simulink model "FlightCore_Gazebo_loop"  (R2025b)
settings: Solver=FixedStepDiscrete  StartTime=0.0  StopTime=(double(GazeboLockstepEpochCount)-1)*GazeboLockstepSampleTime  FixedStep=GazeboLockstepSampleTime  RelTol=1e-3
model workspace (MAT data in the model file):
  GazeboLockstepEpochCount = 20
  GazeboLockstepSampleTime = 0.001
  GazeboLockstepSessionId = 1167057969
  GazeboPrimeTimeoutSec = 300
  GazeboStepResultTimeoutSec = 5
  SL_Bus_ROSEnable64bitIntegers = 1
undefined symbols (not defined in the file): actuator_values, armed, command_id, source_step_id, target_step_id, valid, valid_from_iteration
libraries: ros2lib x4
settings Model: DataDictionary=GlobalTypes.sldd  PacingRate=0.250000  Creator=89447  LastModifiedBy=89447
settings OptimizationCC: DefaultParameterBehavior=Inlined  EnhancedBackFolding=on  PassReuseOutputArgsAs=Individual arguments  ZeroExternalMemoryAtStartup=off  ZeroInternalMemoryAtStartup=off  MaxStackSize=64  OptimizeBlockOrder=speed  DifferentSizesBufferReuse=on  OptimizationCustomize=off  EfficientTunableParamExpr=on
settings HardwareCC: ProdBitPerLong=64.0  ProdHWDeviceType=Intel->x86-64 (Linux 64)
settings SFSimCC: MATLABDynamicMemAlloc=off
settings RTWCC: SystemTargetFile=ert.tlc  HardwareBoard=Robot Operating System 2 (ROS 2)  TLCOptions="-aInlineSetEventsForThisBaseRateFcn=TLC_FALSE -aSuppressMultiTaskScheduler=TLC_FALSE  -aRateBasedStepFcn=0"  GenCodeOnly=on  TemplateMakefile=ert_default_tmf  Toolchain=Colcon Tools  TargetLang=C++  Description=Embedded Coder
settings CodeAppCC: ForceParamTrailComments=on  IgnoreCustomStorageClasses=off  OperatorAnnotations=on  SimulinkDataObjDesc=on  SFDataObjDesc=on  InsertBlockDesc=on
settings ERTTargetCC: ExtModeTransport=2.0  ExtModeStaticAlloc=on  ExtModeAutomaticAllocSize=off  ExtModeMexFile=ext_xcp  ExtModeIntrfLevel=Level2 - Open  RootIOFormat=Structure reference  TargetLangStandard=C++11 (ISO)  CodeInterfacePackaging=C++ class  SupportContinuousTime=on

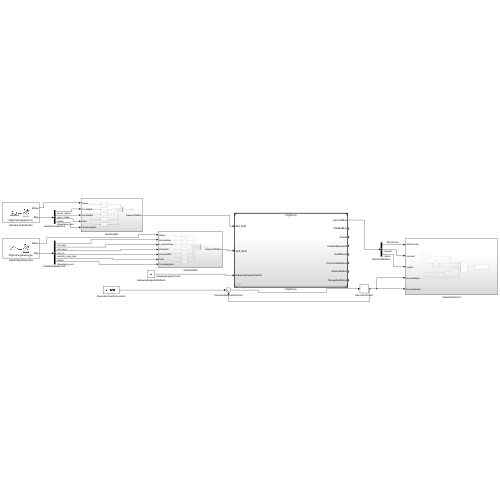
[thumbnail: Simulink's stored preview of the top-level diagram]
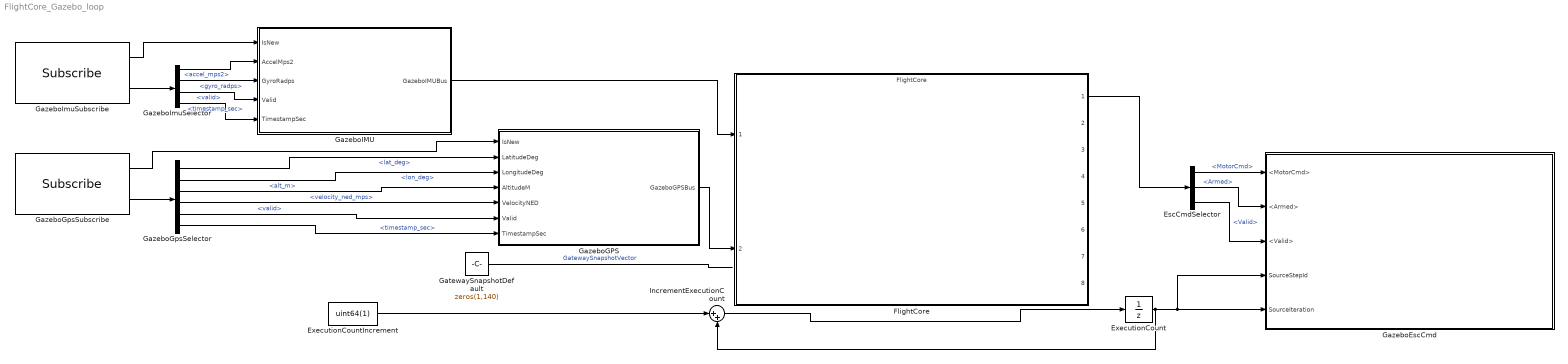
== system FlightCore_Gazebo_loop ==
  EscCmdSelector : BusSelector  OutputSignals=MotorCmd,Armed,Valid
  ExecutionCount : UnitDelay  InitialCondition=uint64(0)  SampleTime=GazeboLockstepSampleTime
  ExecutionCountIncrement : Constant  Value=uint64(1)  SampleTime=GazeboLockstepSampleTime
  FlightCore : ModelReference  ModelNameDialog=FlightCore  SimulationMode=Normal  ModelReferenceVersion=1.37
  GatewaySnapshotDefault : Constant  Value=zeros(1,140)  OutDataTypeStr=double  SampleTime=-1
  GazeboEscCmd : Subsystem
  GazeboGPS : Subsystem
  GazeboGpsSelector : BusSelector  OutputSignals=lat_deg,lon_deg,alt_m,velocity_ned_mps,valid,timestamp_sec
  GazeboGpsSubscribe : ros2lib/Subscribe  topicSource=Specify your own  topic=/flightcore/gazebo/gps  messageType=flightcore_msgs/Gps  sampleTime=GazeboLockstepSampleTime  QOSHistory=Keep last  QOSDepth=10  QOSReliability=Reliable  QOSDurability=Volatile  QOSDeadline=Inf  QOSLifespan=Inf  QOSLiveliness=Automatic  QOSLeaseDuration=Inf  QOSAvoidROSNamespaceConventions=off
  GazeboIMU : Subsystem
  GazeboImuSelector : BusSelector  OutputSignals=accel_mps2,gyro_radps,valid,timestamp_sec
  GazeboImuSubscribe : ros2lib/Subscribe  topicSource=Specify your own  topic=/flightcore/gazebo/imu  messageType=flightcore_msgs/Imu  sampleTime=GazeboLockstepSampleTime  QOSHistory=Keep last  QOSDepth=10  QOSReliability=Reliable  QOSDurability=Volatile  QOSDeadline=Inf  QOSLifespan=Inf  QOSLiveliness=Automatic  QOSLeaseDuration=Inf  QOSAvoidROSNamespaceConventions=off
  IncrementExecutionCount : Sum  Inputs=|++  OutDataTypeStr=uint64
  wires:
  FlightCore/1 -> EscCmdSelector/1
  EscCmdSelector/1 -> GazeboEscCmd/1(<MotorCmd>)  "<MotorCmd>"
  EscCmdSelector/2 -> GazeboEscCmd/2(<Armed>)  "<Armed>"
  GazeboIMU/1(GazeboIMUBus) -> FlightCore/1
  GazeboGPS/1(GazeboGPSBus) -> FlightCore/2
  GazeboImuSubscribe/2 -> GazeboImuSelector/1
  GazeboImuSelector/1 -> GazeboIMU/2(AccelMps2)  "<accel_mps2>"
  GazeboImuSelector/2 -> GazeboIMU/3(GyroRadps)  "<gyro_radps>"
  GazeboImuSelector/3 -> GazeboIMU/4(Valid)  "<valid>"
  GazeboImuSelector/4 -> GazeboIMU/5(TimestampSec)  "<timestamp_sec>"
  GazeboImuSubscribe/1 -> GazeboIMU/1(IsNew)
  GazeboGpsSubscribe/2 -> GazeboGpsSelector/1
  GazeboGpsSelector/1 -> GazeboGPS/2(LatitudeDeg)  "<lat_deg>"
  GazeboGpsSelector/2 -> GazeboGPS/3(LongitudeDeg)  "<lon_deg>"
  GazeboGpsSelector/3 -> GazeboGPS/4(AltitudeM)  "<alt_m>"
  GazeboGpsSelector/4 -> GazeboGPS/5(VelocityNED)  "<velocity_ned_mps>"
  GazeboGpsSelector/5 -> GazeboGPS/6(Valid)  "<valid>"
  GazeboGpsSelector/6 -> GazeboGPS/7(TimestampSec)  "<timestamp_sec>"
  GazeboGpsSubscribe/1 -> GazeboGPS/1(IsNew)
  EscCmdSelector/3 -> GazeboEscCmd/3(<Valid>)  "<Valid>"
  ExecutionCount/1 -> GazeboEscCmd/5(SourceIteration), GazeboEscCmd/4(SourceStepId), IncrementExecutionCount/2
  ExecutionCountIncrement/1 -> IncrementExecutionCount/1
  IncrementExecutionCount/1 -> ExecutionCount/1
  GatewaySnapshotDefault/1 -> ?  "GatewaySnapshotVector"

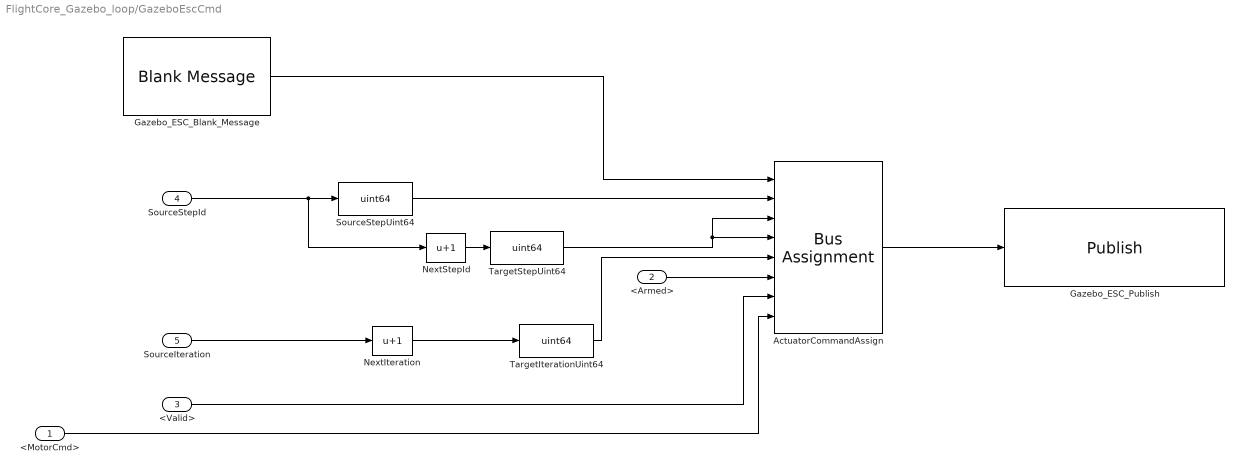
== system FlightCore_Gazebo_loop/GazeboEscCmd ==
  <MotorCmd> : Inport
  <Armed> : Inport  Port=2
  <Valid> : Inport  Port=3
  SourceStepId : Inport  Port=4
  SourceIteration : Inport  Port=5
  ActuatorCommandAssign : BusAssignment  AssignedSignals=source_step_id,target_step_id,command_id,valid_from_iteration,armed,valid,actuator_values
  Gazebo_ESC_Blank_Message : ros2lib/Blank Message  messageClass=Message  entityType=flightcore_gazebo_msgs/ActuatorCommand  messageType=flightcore_gazebo_msgs/ActuatorCommand  SampleTime=inf
  Gazebo_ESC_Publish : ros2lib/Publish  topicSource=Specify your own  topic=/flightcore/gazebo/actuator_command  messageType=flightcore_gazebo_msgs/ActuatorCommand  QOSHistory=Keep last  QOSDepth=1  QOSReliability=Reliable  QOSDurability=Volatile  QOSDeadline=Inf  QOSLifespan=Inf  QOSLiveliness=Automatic  QOSLeaseDuration=Inf  QOSAvoidROSNamespaceConventions=off
  NextIteration : Bias  Bias=1
  NextStepId : Bias  Bias=1
  SourceStepUint64 : DataTypeConversion  OutDataTypeStr=uint64
  TargetIterationUint64 : DataTypeConversion  OutDataTypeStr=uint64
  TargetStepUint64 : DataTypeConversion  OutDataTypeStr=uint64
  wires:
  SourceStepId/1 -> NextStepId/1, SourceStepUint64/1
  NextStepId/1 -> TargetStepUint64/1
  SourceIteration/1 -> NextIteration/1
  NextIteration/1 -> TargetIterationUint64/1
  <Armed>/1 -> ActuatorCommandAssign/6
  <Valid>/1 -> ActuatorCommandAssign/7
  <MotorCmd>/1 -> ActuatorCommandAssign/8
  ActuatorCommandAssign/1 -> Gazebo_ESC_Publish/1
  Gazebo_ESC_Blank_Message/1 -> ActuatorCommandAssign/1
  SourceStepUint64/1 -> ActuatorCommandAssign/2
  TargetStepUint64/1 -> ActuatorCommandAssign/3, ActuatorCommandAssign/4
  TargetIterationUint64/1 -> ActuatorCommandAssign/5

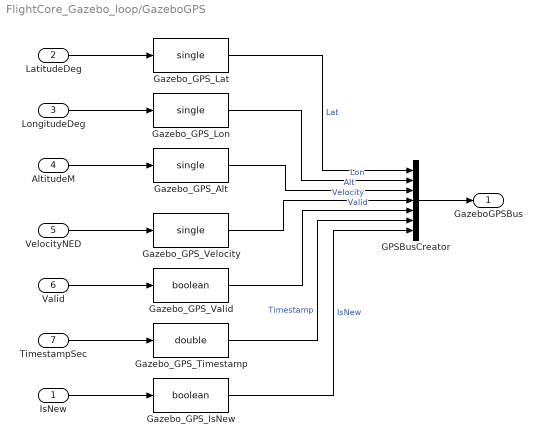
== system FlightCore_Gazebo_loop/GazeboGPS ==
  IsNew : Inport
  LatitudeDeg : Inport  Port=2
  LongitudeDeg : Inport  Port=3
  AltitudeM : Inport  Port=4
  VelocityNED : Inport  Port=5
  Valid : Inport  Port=6
  TimestampSec : Inport  Port=7
  GPSBusCreator : BusCreator  Inputs=7  OutDataTypeStr=Bus: GPS_BUS
  Gazebo_GPS_Alt : DataTypeConversion  OutDataTypeStr=single
  Gazebo_GPS_IsNew : DataTypeConversion  OutDataTypeStr=boolean
  Gazebo_GPS_Lat : DataTypeConversion  OutDataTypeStr=single
  Gazebo_GPS_Lon : DataTypeConversion  OutDataTypeStr=single
  Gazebo_GPS_Timestamp : DataTypeConversion  OutDataTypeStr=double
  Gazebo_GPS_Valid : DataTypeConversion  OutDataTypeStr=boolean
  Gazebo_GPS_Velocity : DataTypeConversion  OutDataTypeStr=single
  GazeboGPSBus : Outport
  wires:
  Gazebo_GPS_Velocity/1 -> GPSBusCreator/4  "Velocity"
  Gazebo_GPS_Valid/1 -> GPSBusCreator/5  "Valid"
  Gazebo_GPS_Lon/1 -> GPSBusCreator/2  "Lon"
  Gazebo_GPS_Lat/1 -> GPSBusCreator/1  "Lat"
  Gazebo_GPS_Timestamp/1 -> GPSBusCreator/6  "Timestamp"
  Gazebo_GPS_Alt/1 -> GPSBusCreator/3  "Alt"
  Gazebo_GPS_IsNew/1 -> GPSBusCreator/7  "IsNew"
  GPSBusCreator/1 -> GazeboGPSBus/1
  LatitudeDeg/1 -> Gazebo_GPS_Lat/1
  LongitudeDeg/1 -> Gazebo_GPS_Lon/1
  AltitudeM/1 -> Gazebo_GPS_Alt/1
  VelocityNED/1 -> Gazebo_GPS_Velocity/1
  Valid/1 -> Gazebo_GPS_Valid/1
  TimestampSec/1 -> Gazebo_GPS_Timestamp/1
  IsNew/1 -> Gazebo_GPS_IsNew/1

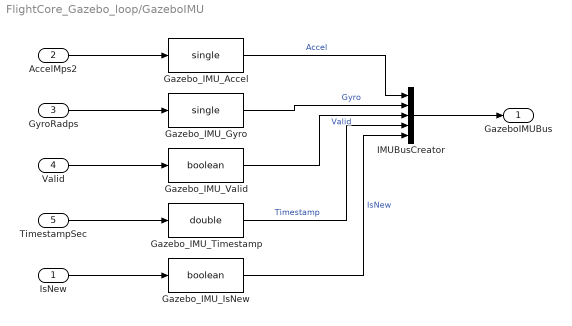
== system FlightCore_Gazebo_loop/GazeboIMU ==
  IsNew : Inport
  AccelMps2 : Inport  Port=2
  GyroRadps : Inport  Port=3
  Valid : Inport  Port=4
  TimestampSec : Inport  Port=5
  Gazebo_IMU_Accel : DataTypeConversion  OutDataTypeStr=single
  Gazebo_IMU_Gyro : DataTypeConversion  OutDataTypeStr=single
  Gazebo_IMU_IsNew : DataTypeConversion  OutDataTypeStr=boolean
  Gazebo_IMU_Timestamp : DataTypeConversion  OutDataTypeStr=double
  Gazebo_IMU_Valid : DataTypeConversion  OutDataTypeStr=boolean
  IMUBusCreator : BusCreator  Inputs=5  OutDataTypeStr=Bus: IMU_BUS
  GazeboIMUBus : Outport
  wires:
  Gazebo_IMU_Timestamp/1 -> IMUBusCreator/4  "Timestamp"
  Gazebo_IMU_IsNew/1 -> IMUBusCreator/5  "IsNew"
  Gazebo_IMU_Accel/1 -> IMUBusCreator/1  "Accel"
  Gazebo_IMU_Valid/1 -> IMUBusCreator/3  "Valid"
  Gazebo_IMU_Gyro/1 -> IMUBusCreator/2  "Gyro"
  IMUBusCreator/1 -> GazeboIMUBus/1
  AccelMps2/1 -> Gazebo_IMU_Accel/1
  GyroRadps/1 -> Gazebo_IMU_Gyro/1
  Valid/1 -> Gazebo_IMU_Valid/1
  TimestampSec/1 -> Gazebo_IMU_Timestamp/1
  IsNew/1 -> Gazebo_IMU_IsNew/1
